simulink subsystem "full_model_robot"  (R2022a)
settings: Solver=VariableStepAuto  StartTime=0.0  StopTime=10.0  RelTol=1e-3
undefined symbols (not defined in the file): hFriction
settings Model: Creator=Philipp  LastModifiedBy=Philipp
settings DebuggingCC: UnconnectedInputMsg=warning  UnconnectedOutputMsg=warning  UnconnectedLineMsg=warning
settings RTWCC: DLArmComputeVersion=19.05

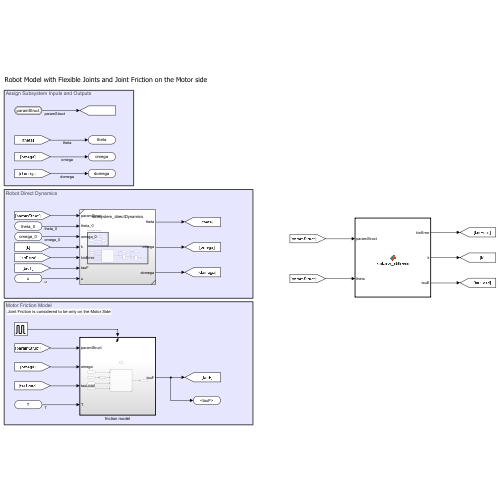
[thumbnail: Simulink's stored preview of the top-level diagram]
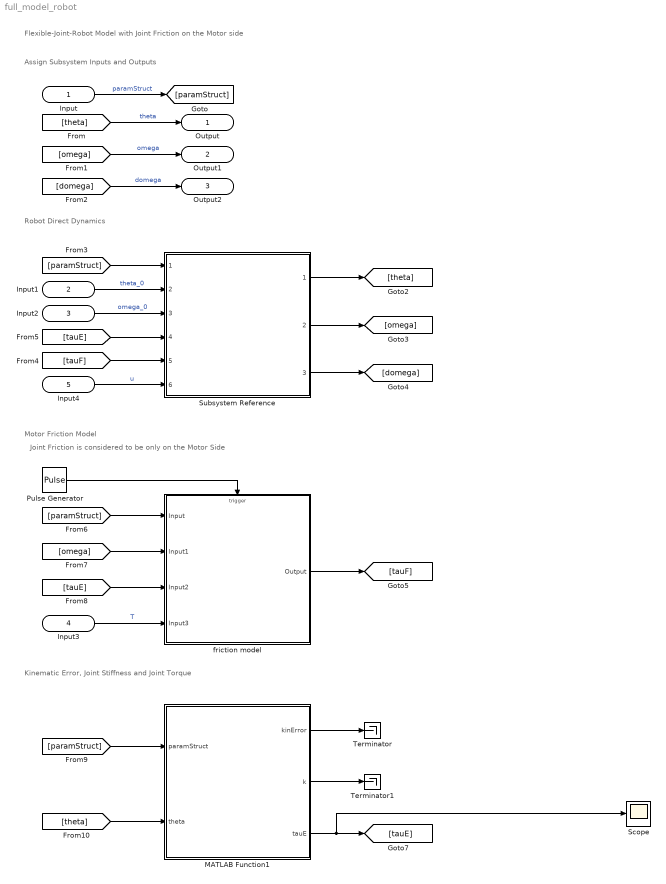
== system full_model_robot ==
  note: Kinematic Error, Joint Stiffness and Joint Torque
  note: Flexible-Joint-Robot Model with Joint Friction on the Motor side
  note: Joint Friction is considered to be only on the Motor Side
  note: Motor Friction Model
  note: Robot Direct Dynamics
  note: Assign Subsystem Inputs and Outputs
  Input : Inport  OutDataTypeStr=Bus: main_bus
  Input1 : Inport  Port=2  PortDimensions=6
  Input2 : Inport  Port=3  PortDimensions=6
  Input3 : Inport  Port=4
  Input4 : Inport  Port=5  PortDimensions=3
  MATLAB Function1 : MATLAB Function  TreatAsAtomicUnit=on
  Pulse Generator : DiscretePulseGenerator  PulseType=Time based  Period=hFriction  PulseWidth=5
  Scope : Scope
  Subsystem Reference : Subsystem  ReferencedSubsystem=subsystem_directDynamics
  Terminator : Terminator
  Terminator1 : Terminator
  friction model : Subsystem  TreatAsAtomicUnit=on
  Output : Outport  PortDimensions=6
  Output1 : Outport  Port=2  PortDimensions=6
  Output2 : Outport  Port=3  PortDimensions=6
  wires:
  Input/1 -> [paramStruct]  "paramStruct"
  [theta] -> Output/1  "theta"
  [domega] -> Output2/1  "domega"
  [omega] -> Output1/1  "omega"
  Input1/1 -> Subsystem Reference/2  "theta_0"
  [paramStruct] -> Subsystem Reference/1
  Input2/1 -> Subsystem Reference/3  "omega_0"
  Subsystem Reference/1 -> [theta]
  Subsystem Reference/3 -> [domega]
  Subsystem Reference/2 -> [omega]
  Pulse Generator/1 -> friction model/Trigger
  [paramStruct] -> friction model/1(Input)
  [omega] -> friction model/2(Input1)
  Input3/1 -> friction model/4(Input3)  "T"
  [tauE] -> friction model/3(Input2)
  friction model/1(Output) -> [tauF]
  [tauE] -> Subsystem Reference/4
  [paramStruct] -> MATLAB Function1/1(paramStruct)
  [theta] -> MATLAB Function1/2(theta)
  MATLAB Function1/2(k) -> Terminator1/1
  MATLAB Function1/1(kinError) -> Terminator/1
  MATLAB Function1/3(tauE) -> [tauE], Scope/1
  Input4/1 -> Subsystem Reference/6  "u"
  [tauF] -> Subsystem Reference/5

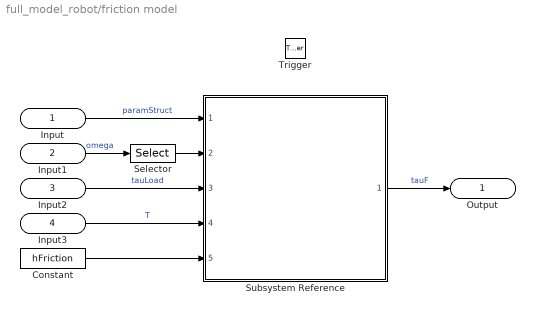
== system full_model_robot/friction model ==
  Input : Inport  OutDataTypeStr=Bus: main_bus
  Input1 : Inport  Port=2
  Input2 : Inport  Port=3
  Input3 : Inport  Port=4
  Trigger : TriggerPort  VariantControl=(inherit)
  Constant : Constant  Value=hFriction
  Selector : Selector  InputPortWidth=6  IndexOptions=Index vector (dialog)  Indices=4:6  OutputSizes=1
  Subsystem Reference : Subsystem  ReferencedSubsystem=subsystem_lugreFriction
  Output : Outport
  wires:
  Constant/1 -> Subsystem Reference/5
  Subsystem Reference/1 -> Output/1  "tauF"
  Selector/1 -> Subsystem Reference/2
  Input1/1 -> Selector/1  "omega"
  Input2/1 -> Subsystem Reference/3  "tauLoad"
  Input3/1 -> Subsystem Reference/4  "T"
  Input/1 -> Subsystem Reference/1  "paramStruct"

== matlab function full_model_robot/MATLAB Function1 ==
  data: paramStruct input; theta input; kinError output; k output; tauE output
function [kinError, k, tauE] = kinError_stiffness(paramStruct, theta)

% Convert to deg
thetaDeg = theta .* (180/pi);

% Calculate kinematic error
%kinErrorDeg = kinError_fun(paramStruct, thetaDeg(4:6));
kinErrorDeg = zeros(3,1); % Do not consider in model because it results in sigularities for numerical integration

% Calculate stiffness
[thetaDiffE, ~] = compKinError_fun(thetaDeg, zeros(6,1), kinErrorDeg, zeros(3,1));
kDeg = stiffness_fun(paramStruct, thetaDiffE);

% Calculate stiffness torque
[tauE, ~] = stiffnessTorque_fun(kDeg, thetaDiffE, zeros(3,1));

% Convert to rad
kinError = kinErrorDeg .* (pi/180);
k = kDeg .* (180/pi);
